simulink model "lab5sim"  (R2022b)
settings: Solver=VariableStepAuto  StartTime=0.0  StopTime=10.0  RelTol=1e-3
values from neighbouring files (symbols this model uses):
  dqg = 100    [lab5_przygotowanie.m]
  dTzew = 0    [lab5_przygotowanie.m]
  L11 = [Cvp, kcwp+kcp]    [lab5_przygotowanie.m]
  L12 = [Cvp*kcw, kcwp*kcp+kcwp*kcw+kcp*kcw]    [lab5_przygotowanie.m]
  L21 = [0, kcwp]    [lab5_przygotowanie.m]
  L22 = [Cvw*kcp, kcwp*kcw+kcw*kcp+kcwp*kcp]    [lab5_przygotowanie.m]
  M = [Cvw*Cvp, Cvw*kcwp+Cvw*kcp+Cvp*kcw, kcw*kcwp+kcp*kcw]    [lab5_przygotowanie.m]
  t0 = 1000    [lab5_przygotowanie.m]
  Tp0 = ((kcp*Tzew0)*(kcw+kcwp)+kcwp*(qg0+kcw*Tzew0))/(kcwp*kcw+kcp*kcw+kcp*kcwp)    (= 10)    [lab5_przygotowanie.m]
  Twew0 = (qg0+kcw*Tzew0+kcwp*Tp0)/(kcw+kcwp)    (= 20)    [lab5_przygotowanie.m]
settings Model: Creator=Dawid  LastModifiedBy=Dawid
settings DataIOCC: ReturnWorkspaceOutputs=off

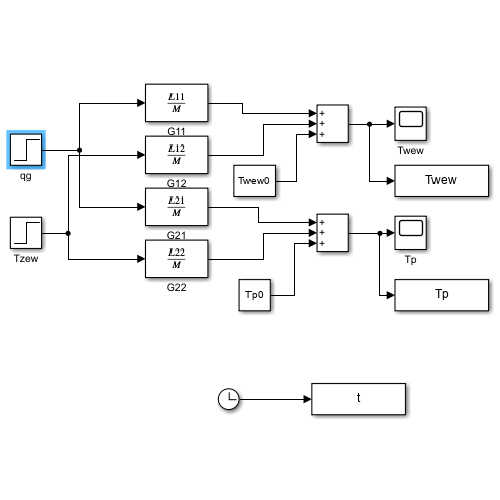
[thumbnail: Simulink's stored preview of the top-level diagram]
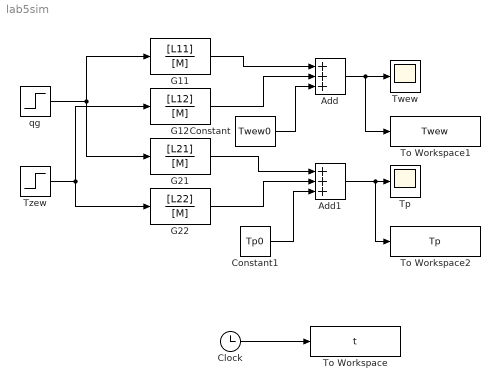
== system lab5sim ==
  Add : Sum  Inputs=+++
  Add1 : Sum  Inputs=+++
  Clock : Clock
  Constant : Constant  Value=Twew0
  Constant1 : Constant  Value=Tp0
  G11 : TransferFcn  Numerator=[L11]  Denominator=[M]
  G12 : TransferFcn  Numerator=[L12]  Denominator=[M]
  G21 : TransferFcn  Numerator=[L21]  Denominator=[M]
  G22 : TransferFcn  Numerator=[L22]  Denominator=[M]
  To Workspace : ToWorkspace  VariableName=t  SaveFormat=Timeseries  SampleTime=-1
  To Workspace1 : ToWorkspace  VariableName=Twew  SampleTime=-1
  To Workspace2 : ToWorkspace  VariableName=Tp  SampleTime=-1
  Tp : Scope
  Twew : Scope
  Tzew : Step  Time=t0  After=dTzew  SampleTime=0
  qg : Step  Time=t0  After=dqg  SampleTime=0
  wires:
  Add/1 -> To Workspace1/1, Twew/1
  Add1/1 -> To Workspace2/1, Tp/1
  qg/1 -> G21/1, G11/1
  Tzew/1 -> G22/1, G12/1
  G11/1 -> Add/1
  G12/1 -> Add/2
  G21/1 -> Add1/1
  G22/1 -> Add1/2
  Constant/1 -> Add/3
  Constant1/1 -> Add1/3
  Clock/1 -> To Workspace/1
